simulink model "fangzhen20050606"  (Simulink 9.0)
settings: Solver=ode4  StartTime=0.0  StopTime=1200.0  FixedStep=0.05  RelTol=1e-3
InitFcn:
  | data
values from neighbouring files (symbols this model uses):
  A = [1    0     0 ... (first row only)    [cx.m]    (also in data.m = [Wex^2-W^2   Wex*Wey    Wex*Wez; data1.m = [Wex^2-W^2   Wex*Wey    Wex*Wez)
  a = F/m0    (= 0.2)    [data.m]    (also in data1.m = 0.02)
  a0 = 2*a*k/(4*a+k)    (= 0.08)    [data.m]    (also in data1.m = 0.00363636363636)
  AWcc = [1 1 1]*0.15/3600/3*pi/180    [data.m]    (also in data1.m)
  B = [   0    -2*Wez    2*Wey ... (first row only)    [data.m]    (also in data1.m)
  b = 0.00001*(a+a0)/(2*a*a0)    (= 8.75e-05)    [data.m]    (also in data1.m = 0.01625)
  c20 = -0.113    [data.m]    (also in data1.m)
  c22 = 0.0396    [data.m]    (also in data1.m)
  CWw = [1,1,1,1]*6e-5    [data.m]    (also in data1.m)
  d = 0.01    [data.m]    (also in data1.m = 0.1)
  DWN = [sin(bata)*cos(alpha)  sin(bata)*sin(alpha)  -sin(bata)*cos(alpha)  -sin(bata)*sin(alpha) ... (first row only)    [data.m]    (also in data1.m)
  F = 40    [data.m]    (also in data1.m = 4)
  f = f+2*pi    [E2C.m]    (also in data.m = -0.02; data1.m = 0.02)
  Gl = [-cos(xit0)*sin(fai0)   sin(xit0)*sin(fai0)    cos(fai0) ... (first row only)    [data.m]    (also in data1.m)
  HBd0 = IBd*We0    [data.m]    (also in data1.m)
  Hwmax = JW.*Wwmax    [data.m]    (also in data1.m)
  HWw0 = [0.01 0.01 0.01 0.01]    [data.m]    (also in data1.m)
  InvIBd = inv(IBd)    [data.m]    (also in data1.m)
  invJW = 1 ./JW    [data.m]    (also in data1.m)
  Isp = 300*9.8    (= 2940)    [data.m]    (also in data1.m)
  IW = [1,1,1,1]*1.e-6    [data.m]    (also in data1.m)
  JW = [1,1,1,1]*0.0017362    [data.m]    (also in data1.m)
  Kd = [19.2895;16.6643;22.1166]    [data.m]    (also in data1.m)
  Ki = [0.0503;0.0503;0.0503]    [data.m]    (also in data1.m)
  Kp = [7.0313;6.0484;8.0898]    [data.m]    (also in data1.m)
  m0 = 200    [data.m]    (also in data1.m)
  Mu = 4.794e3    (= 4794)    [data.m]    (also in data1.m)
  MWN = DWN'*inv(DWN*DWN')    [data.m]    (also in data1.m)
  Noise_gc = [1 -1 1]*6/3600*pi/180    [data.m]    (also in data1.m)
  Noise_gn = ([1 1 1]*0.0025/3.*pi/180).^2    [data.m]    (also in data1.m)
  Noise_rwn = ([1 1 1].*1e-10).^2    [data.m]    (also in data1.m)
  Qb0 = [QQQ(4);QQQ(1:3)]    [data.m]    (also in data1.m)
  r0 = [100;-200;1000]    [data.m]    (also in data1.m = [200;300;1000])
  R0 = Tl*[0;0;R0l]    [data.m]    (also in data1.m)
  re = 1750    [data.m]    (also in data1.m)
  rg0 = [3;-104;950]    [data.m]    (also in data1.m = [203;292;998])
  Rtb = [0;0;0]    [data.m]    (also in data1.m = [-30;50;0])
  T = 200    [data.m]    (also in data1.m = 1200)
  TA = [0 0 0]'    [data.m]    (also in data1.m)
  TB = [500 0 0]'    [data.m]    (also in data1.m)
  TC = [500 500 0]'    [data.m]    (also in data1.m)
  Tcmax = [1,1,1,1].*0.02    [data.m]    (also in data1.m)
  TWf0 = [1,1,1,1]*3e-4    [data.m]    (also in data1.m)
  v0 = [-0.1;0.1;-0.3]    [data.m]    (also in data1.m = [0.1;0.1;-1.0])
  vg0 = [0;-0.1;-0.4]    [data.m]    (also in data1.m = [0;-0.1;-0.7])
  Wcc = [1 1 1]*0.2    [data.m]    (also in data1.m)
  We = Tl*Gl'*[0;0;W]    [data.m]    (also in data1.m)
  Wgmax = 10*[1,1,1]'*pi/180    [data.m]    (also in data1.m)
undefined symbols (not defined in the file or in its folder): DiscIntNeverNeededParam, HB0, magnitude
libraries: sharedtransform x4, aerolibobsolete x4, sharedutil x1
(part 2 of 2)

== system fangzhen20050606/GNC System/轨迹制导0515(2)1/轨迹制导2/r ==
  tgo : Inport
  t : Inport  Port=2
  r0 : Inport  Port=3
  v0 : Inport  Port=4
  Gain1 : Gain  Gain=-2  SaturateOnIntegerOverflow=on  OutDataTypeStr=Inherit: Same as input  ParamDataTypeStr=Inherit: Same as input
  Gain2 : Gain  Gain=2  SaturateOnIntegerOverflow=on  OutDataTypeStr=Inherit: Same as input  ParamDataTypeStr=Inherit: Same as input
  Gain4 : Gain  Gain=-3  SaturateOnIntegerOverflow=on  OutDataTypeStr=Inherit: Same as input  ParamDataTypeStr=Inherit: Same as input
  Math Function1 : Math  Operator=magnitude^2  SaturateOnIntegerOverflow=on
  Math Function2 : Math  Operator=magnitude^2  SaturateOnIntegerOverflow=on
  Product{1..2,4,7..8} (5 alike) : Product  Inputs=**  SaturateOnIntegerOverflow=on  OutDataTypeStr=Inherit: Same as first input
  Product3 : Product  Inputs=**/  SaturateOnIntegerOverflow=on  OutDataTypeStr=Inherit: Same as first input
  Product6 : Product  Inputs=**/  SaturateOnIntegerOverflow=on  OutDataTypeStr=Inherit: Same as first input
  Sum1 : Sum  Inputs=++++  SaturateOnIntegerOverflow=on
  Sum2 : Sum  SaturateOnIntegerOverflow=on
  Sum3 : Sum  SaturateOnIntegerOverflow=on
  r : Outport
  wires:
  Product6/1 -> Sum1/2
  Product8/1 -> Product6/1
  Product7/1 -> Product6/3
  Sum3/1 -> Product6/2
  Product4/1 -> Sum3/1
  Gain2/1 -> Sum3/2
  Product3/1 -> Sum1/3
  Math Function1/1 -> Product8/2, Product3/1
  Sum2/1 -> Product3/2
  Math Function2/1 -> Product7/1, Product3/3
  Gain4/1 -> Sum2/2
  Gain1/1 -> Sum2/1
  Product2/1 -> Gain1/1
  tgo/1 -> Product7/2, Math Function2/1, Product4/2, Product2/2
  Product1/1 -> Sum1/1
  r0/1 -> Gain2/1, Sum1/4, Gain4/1
  v0/1 -> Product4/1, Product2/1, Product1/2
  t/1 -> Product8/1, Math Function1/1, Product1/1
  Sum1/1 -> r/1

== system fangzhen20050606/GNC System/轨迹制导0515(2)1/轨迹制导2/v ==
  tgo : Inport
  t : Inport  Port=2
  r0 : Inport  Port=3
  v0 : Inport  Port=4
  Gain1 : Gain  Gain=-6  SaturateOnIntegerOverflow=on  OutDataTypeStr=Inherit: Same as input  ParamDataTypeStr=Inherit: Same as input
  Gain2 : Gain  Gain=-4  SaturateOnIntegerOverflow=on  OutDataTypeStr=Inherit: Same as input  ParamDataTypeStr=Inherit: Same as input
  Gain4 : Gain  Gain=6  SaturateOnIntegerOverflow=on  OutDataTypeStr=Inherit: Same as input  ParamDataTypeStr=Inherit: Same as input
  Gain5 : Gain  Gain=3  SaturateOnIntegerOverflow=on  OutDataTypeStr=Inherit: Same as input  ParamDataTypeStr=Inherit: Same as input
  Math Function1 : Math  Operator=magnitude^2  SaturateOnIntegerOverflow=on
  Math Function4 : Math  Operator=magnitude^2  SaturateOnIntegerOverflow=on
  Product1 : Product  Inputs=**  SaturateOnIntegerOverflow=on  OutDataTypeStr=Inherit: Same as first input
  Product2 : Product  Inputs=**/  SaturateOnIntegerOverflow=on  OutDataTypeStr=Inherit: Same as first input
  Product5 : Product  Inputs=**/  SaturateOnIntegerOverflow=on  OutDataTypeStr=Inherit: Same as first input
  Product9 : Product  Inputs=**  SaturateOnIntegerOverflow=on  OutDataTypeStr=Inherit: Same as first input
  Sum1 : Sum  Inputs=+++  SaturateOnIntegerOverflow=on
  Sum2 : Sum  SaturateOnIntegerOverflow=on
  Sum3 : Sum  SaturateOnIntegerOverflow=on
  v : Outport
  wires:
  Product2/1 -> Sum1/1
  Product9/1 -> Product2/3
  Math Function1/1 -> Product2/1
  Sum3/1 -> Product2/2
  Gain4/1 -> Sum3/2
  Gain5/1 -> Sum3/1
  Product5/1 -> Sum1/2
  Math Function4/1 -> Product9/2, Product5/3
  t/1 -> Math Function1/1, Product5/1
  Sum2/1 -> Product5/2
  Gain2/1 -> Sum2/1
  Product1/1 -> Gain5/1, Gain2/1
  tgo/1 -> Product9/1, Math Function4/1, Product1/1
  Gain1/1 -> Sum2/2
  r0/1 -> Gain4/1, Gain1/1
  v0/1 -> Product1/2, Sum1/3
  Sum1/1 -> v/1

== system fangzhen20050606/GNC System/轨迹制导0515(2)1/轨迹制导4/C0 ==
  r : Inport
  v : Inport  Port=2
  tgo : Inport  Port=3
  rt : Inport  Port=4
  Gain : Gain  Gain=-6  SaturateOnIntegerOverflow=on  OutDataTypeStr=Inherit: Same as input  ParamDataTypeStr=Inherit: Same as input
  Gain1 : Gain  Gain=-12  SaturateOnIntegerOverflow=on  OutDataTypeStr=Inherit: Same as input  ParamDataTypeStr=Inherit: Same as input
  Math Function : Math  Operator=magnitude^2  SaturateOnIntegerOverflow=on
  Product : Product  Inputs=*/  SaturateOnIntegerOverflow=on  OutDataTypeStr=Inherit: Same as first input
  Product1 : Product  Inputs=*/  SaturateOnIntegerOverflow=on  OutDataTypeStr=Inherit: Same as first input
  Sum : Sum  SaturateOnIntegerOverflow=on
  Sum1 : Sum  Inputs=+-  SaturateOnIntegerOverflow=on
  C0 : Outport
  wires:
  tgo/1 -> Math Function/1, Product1/2
  v/1 -> Product1/1
  Product1/1 -> Gain/1
  Math Function/1 -> Product/2
  Product/1 -> Gain1/1
  Gain1/1 -> Sum/2
  Gain/1 -> Sum/1
  Sum/1 -> C0/1
  Sum1/1 -> Product/1
  r/1 -> Sum1/1
  rt/1 -> Sum1/2

== system fangzhen20050606/GNC System/轨迹制导0515(2)1/轨迹制导4/C1 ==
  r : Inport
  v : Inport  Port=2
  tgo : Inport  Port=3
  rt : Inport  Port=4
  Gain2 : Gain  Gain=18  SaturateOnIntegerOverflow=on  OutDataTypeStr=Inherit: Same as input  ParamDataTypeStr=Inherit: Same as input
  Gain3 : Gain  Gain=48  SaturateOnIntegerOverflow=on  OutDataTypeStr=Inherit: Same as input  ParamDataTypeStr=Inherit: Same as input
  Math Function1 : Math  Operator=magnitude^2  SaturateOnIntegerOverflow=on
  Product2 : Product  Inputs=*/  SaturateOnIntegerOverflow=on  OutDataTypeStr=Inherit: Same as first input
  Product3 : Product  Inputs=**  SaturateOnIntegerOverflow=on  OutDataTypeStr=Inherit: Same as first input
  Product4 : Product  Inputs=/*  SaturateOnIntegerOverflow=on  OutDataTypeStr=Inherit: Same as first input
  Sum1 : Sum  SaturateOnIntegerOverflow=on
  Sum2 : Sum  Inputs=+-  SaturateOnIntegerOverflow=on
  C1 : Outport
  wires:
  tgo/1 -> Math Function1/1, Product3/2
  Math Function1/1 -> Product2/2, Product3/1
  v/1 -> Product2/1
  Product2/1 -> Gain2/1
  Product3/1 -> Product4/1
  Product4/1 -> Gain3/1
  Sum1/1 -> C1/1
  Gain3/1 -> Sum1/2
  Gain2/1 -> Sum1/1
  Sum2/1 -> Product4/2
  r/1 -> Sum2/1
  rt/1 -> Sum2/2

== system fangzhen20050606/GNC System/轨迹制导0515(2)1/轨迹制导4/C2 ==
  r : Inport
  v : Inport  Port=2
  tgo : Inport  Port=3
  rt : Inport  Port=4
  Gain2 : Gain  Gain=-12  SaturateOnIntegerOverflow=on  OutDataTypeStr=Inherit: Same as input  ParamDataTypeStr=Inherit: Same as input
  Gain3 : Gain  Gain=-36  SaturateOnIntegerOverflow=on  OutDataTypeStr=Inherit: Same as input  ParamDataTypeStr=Inherit: Same as input
  Math Function1 : Math  Operator=magnitude^2  SaturateOnIntegerOverflow=on
  Product2 : Product  Inputs=*/  SaturateOnIntegerOverflow=on  OutDataTypeStr=Inherit: Same as first input
  Product3 : Product  Inputs=**  SaturateOnIntegerOverflow=on  OutDataTypeStr=Inherit: Same as first input
  Product4 : Product  Inputs=**  SaturateOnIntegerOverflow=on  OutDataTypeStr=Inherit: Same as first input
  Product5 : Product  Inputs=/*  SaturateOnIntegerOverflow=on  OutDataTypeStr=Inherit: Same as first input
  Sum1 : Sum  SaturateOnIntegerOverflow=on
  Sum2 : Sum  Inputs=+-  SaturateOnIntegerOverflow=on
  C2 : Outport
  wires:
  tgo/1 -> Math Function1/1, Product3/2
  Math Function1/1 -> Product3/1, Product4/1, Product4/2
  Product3/1 -> Product2/2
  v/1 -> Product2/1
  Product2/1 -> Gain2/1
  Product4/1 -> Product5/1
  Product5/1 -> Gain3/1
  Gain3/1 -> Sum1/2
  Gain2/1 -> Sum1/1
  Sum1/1 -> C2/1
  rt/1 -> Sum2/2
  Sum2/1 -> Product5/2
  r/1 -> Sum2/1

== system fangzhen20050606/GNC System/轨迹制导0515(2)1/轨迹制导4/r ==
  C0 : Inport
  C1 : Inport  Port=2
  C2 : Inport  Port=3
  t : Inport  Port=4
  r0 : Inport  Port=5
  v0 : Inport  Port=6
  Gain1 : Gain  Gain=0.5  SaturateOnIntegerOverflow=on  OutDataTypeStr=Inherit: Same as input  ParamDataTypeStr=Inherit: Same as input
  Gain2 : Gain  Gain=1/12  SaturateOnIntegerOverflow=on  OutDataTypeStr=Inherit: Same as input  ParamDataTypeStr=Inherit: Same as input
  Gain3 : Gain  Gain=1/6  SaturateOnIntegerOverflow=on  OutDataTypeStr=Inherit: Same as input  ParamDataTypeStr=Inherit: Same as input
  Math Function1 : Math  Operator=magnitude^2  SaturateOnIntegerOverflow=on
  Product{1..4,6..7} (6 alike) : Product  Inputs=**  SaturateOnIntegerOverflow=on  OutDataTypeStr=Inherit: Same as first input
  Sum1 : Sum  Inputs=+++++  SaturateOnIntegerOverflow=on
  r : Outport
  wires:
  t/1 -> Math Function1/1, Product2/2, Product7/1
  C0/1 -> Product3/1
  C1/1 -> Product1/1
  Product1/1 -> Gain3/1
  Math Function1/1 -> Product3/2, Product2/1, Product4/1, Product4/2
  Product3/1 -> Gain1/1
  Product2/1 -> Product1/2
  C2/1 -> Product6/1
  Product4/1 -> Product6/2
  Product6/1 -> Gain2/1
  v0/1 -> Product7/2
  Gain1/1 -> Sum1/1
  Gain3/1 -> Sum1/2
  Gain2/1 -> Sum1/3
  Product7/1 -> Sum1/4
  r0/1 -> Sum1/5
  Sum1/1 -> r/1

== system fangzhen20050606/GNC System/轨迹制导0515(2)1/轨迹制导4/v ==
  C0 : Inport
  C1 : Inport  Port=2
  C2 : Inport  Port=3
  t : Inport  Port=4
  v0 : Inport  Port=5
  Gain1 : Gain  Gain=1/3  SaturateOnIntegerOverflow=on  OutDataTypeStr=Inherit: Same as input  ParamDataTypeStr=Inherit: Same as input
  Gain3 : Gain  Gain=0.5  SaturateOnIntegerOverflow=on  OutDataTypeStr=Inherit: Same as input  ParamDataTypeStr=Inherit: Same as input
  Math Function1 : Math  Operator=magnitude^2  SaturateOnIntegerOverflow=on
  Product{1,3..5} (4 alike) : Product  Inputs=**  SaturateOnIntegerOverflow=on  OutDataTypeStr=Inherit: Same as first input
  Sum1 : Sum  Inputs=++++  SaturateOnIntegerOverflow=on
  v : Outport
  wires:
  C0/1 -> Product3/1
  t/1 -> Product3/2, Math Function1/1, Product5/2
  Math Function1/1 -> Product1/2, Product5/1
  C1/1 -> Product1/1
  Product1/1 -> Gain3/1
  C2/1 -> Product4/1
  Product5/1 -> Product4/2
  Product4/1 -> Gain1/1
  Product3/1 -> Sum1/1
  Gain3/1 -> Sum1/2
  Gain1/1 -> Sum1/3
  v0/1 -> Sum1/4
  Sum1/1 -> v/1

== system fangzhen20050606/Dynamics System动力系统/Attitude姿态/反作用飞轮/Torque/3x3 Cross Product ==
  A : Inport
  B : Inport  Port=2
  Product : Product  SaturateOnIntegerOverflow=on  InputSameDT=on  OutDataTypeStr=Inherit: Same as first input
  Product1 : Product  SaturateOnIntegerOverflow=on  InputSameDT=on  OutDataTypeStr=Inherit: Same as first input
  Selector : Selector  InputPortWidth=3  IndexOptions=Index vector (dialog)  Indices=[2 3 1]  OutputSizes=1
  Selector1 : Selector  InputPortWidth=3  IndexOptions=Index vector (dialog)  Indices=[3 1 2]  OutputSizes=1
  Selector2 : Selector  InputPortWidth=3  IndexOptions=Index vector (dialog)  Indices=[2 3 1]  OutputSizes=1
  Selector3 : Selector  InputPortWidth=3  IndexOptions=Index vector (dialog)  Indices=[3 1 2]  OutputSizes=1
  Sum : Sum  Inputs=+|-  SaturateOnIntegerOverflow=on  InputSameDT=on  OutDataTypeStr=Inherit: Same as first input
  C : Outport  InitialOutput=0
  wires:
  Sum/1 -> C/1
  B/1 -> Selector1/1, Selector2/1
  Selector/1 -> Product/1
  A/1 -> Selector/1, Selector3/1
  Product/1 -> Sum/1
  Selector1/1 -> Product/2
  Product1/1 -> Sum/2
  Selector2/1 -> Product1/2
  Selector3/1 -> Product1/1

== system fangzhen20050606/Dynamics System动力系统/Orbit轨道/轨道动力学模型/小行星引力加速度/小行星引力 ==
  note: z'
  note: y'
  note: x'
  r' : Inport
  Demux : Demux  Outputs=3
  K : Subsystem
  L : Subsystem
  Mux : Mux  Inputs=3
  Ux : Subsystem
  Uy : Subsystem
  Uz : Subsystem
  rt : Subsystem
  U : Outport
  wires:
  Demux/1 -> Ux/1(x'), L/2(x')
  r'/1 -> Demux/1, rt/1(r')
  Mux/1 -> U/1
  Uy/1(Uy) -> Mux/2
  Ux/1(Ux) -> Mux/1
  Uz/1(Uz) -> Mux/3
  rt/1(rt) -> Ux/2(rt), Uz/2(rt), K/2(rt), Uy/2(rt)
  Demux/3 -> Uz/1(z'), K/1(z')
  Demux/2 -> Uy/1(y'), L/1(y')
  K/1(K) -> Uz/4(K), Ux/4(K), Uy/4(K)
  L/1(L) -> Uz/3(L), Ux/3(L), Uy/3(L)

== system fangzhen20050606/GNC System/导航与滤波/Calculate/Subsystem3/e2 ==
  A : Inport
  B : Inport  Port=2
  Product : Product  SaturateOnIntegerOverflow=on  InputSameDT=on  OutDataTypeStr=Inherit: Same as first input
  Product1 : Product  SaturateOnIntegerOverflow=on  InputSameDT=on  OutDataTypeStr=Inherit: Same as first input
  Selector : Selector  InputPortWidth=3  IndexOptions=Index vector (dialog)  Indices=[2 3 1]  OutputSizes=1
  Selector1 : Selector  InputPortWidth=3  IndexOptions=Index vector (dialog)  Indices=[3 1 2]  OutputSizes=1
  Selector2 : Selector  InputPortWidth=3  IndexOptions=Index vector (dialog)  Indices=[2 3 1]  OutputSizes=1
  Selector3 : Selector  InputPortWidth=3  IndexOptions=Index vector (dialog)  Indices=[3 1 2]  OutputSizes=1
  Sum : Sum  Inputs=+|-  SaturateOnIntegerOverflow=on  InputSameDT=on  OutDataTypeStr=Inherit: Same as first input
  C : Outport  InitialOutput=0
  wires:
  Sum/1 -> C/1
  B/1 -> Selector1/1, Selector2/1
  Selector/1 -> Product/1
  A/1 -> Selector/1, Selector3/1
  Product/1 -> Sum/1
  Selector1/1 -> Product/2
  Product1/1 -> Sum/2
  Selector2/1 -> Product1/2
  Selector3/1 -> Product1/1

== system fangzhen20050606/GNC System/导航与滤波/Calculate/Subsystem3/e4 ==
  A : Inport
  B : Inport  Port=2
  Product : Product  SaturateOnIntegerOverflow=on  InputSameDT=on  OutDataTypeStr=Inherit: Same as first input
  Product1 : Product  SaturateOnIntegerOverflow=on  InputSameDT=on  OutDataTypeStr=Inherit: Same as first input
  Selector : Selector  InputPortWidth=3  IndexOptions=Index vector (dialog)  Indices=[2 3 1]  OutputSizes=1
  Selector1 : Selector  InputPortWidth=3  IndexOptions=Index vector (dialog)  Indices=[3 1 2]  OutputSizes=1
  Selector2 : Selector  InputPortWidth=3  IndexOptions=Index vector (dialog)  Indices=[2 3 1]  OutputSizes=1
  Selector3 : Selector  InputPortWidth=3  IndexOptions=Index vector (dialog)  Indices=[3 1 2]  OutputSizes=1
  Sum : Sum  Inputs=+|-  SaturateOnIntegerOverflow=on  InputSameDT=on  OutDataTypeStr=Inherit: Same as first input
  C : Outport  InitialOutput=0
  wires:
  Selector3/1 -> Product1/1
  Selector2/1 -> Product1/2
  Product1/1 -> Sum/2
  Selector1/1 -> Product/2
  Product/1 -> Sum/1
  A/1 -> Selector3/1, Selector/1
  Selector/1 -> Product/1
  B/1 -> Selector2/1, Selector1/1
  Sum/1 -> C/1

== system fangzhen20050606/Dynamics System动力系统/Orbit轨道/轨道动力学模型/小行星引力加速度/小行星引力/K ==
  z' : Inport
  rt : Inport  Port=2
  Product : Product  Inputs=*/  SaturateOnIntegerOverflow=on  OutDataTypeStr=Inherit: Same as first input
  Trigonometric Function : Trigonometry  Operator=asin
  K : Outport
  wires:
  Trigonometric Function/1 -> K/1
  z'/1 -> Product/1
  rt/1 -> Product/2
  Product/1 -> Trigonometric Function/1

== system fangzhen20050606/Dynamics System动力系统/Orbit轨道/轨道动力学模型/小行星引力加速度/小行星引力/L ==
  y' : Inport
  x' : Inport  Port=2
  Product : Product  Inputs=*/  SaturateOnIntegerOverflow=on  OutDataTypeStr=Inherit: Same as first input
  Trigonometric Function : Trigonometry  Operator=atan
  L : Outport
  wires:
  Product/1 -> Trigonometric Function/1
  y'/1 -> Product/1
  x'/1 -> Product/2
  Trigonometric Function/1 -> L/1

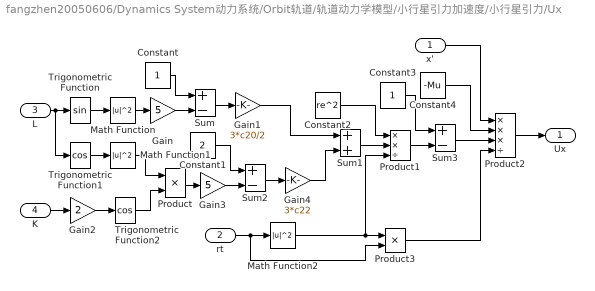
== system fangzhen20050606/Dynamics System动力系统/Orbit轨道/轨道动力学模型/小行星引力加速度/小行星引力/Ux ==
  x' : Inport
  rt : Inport  Port=2
  L : Inport  Port=3
  K : Inport  Port=4
  Constant : Constant
  Constant1 : Constant  Value=2
  Constant2 : Constant  Value=re^2
  Constant3 : Constant
  Constant4 : Constant  Value=-Mu
  Gain : Gain  Gain=5  SaturateOnIntegerOverflow=on  OutDataTypeStr=Inherit: Same as input  ParamDataTypeStr=Inherit: Same as input
  Gain1 : Gain  Gain=3*c20/2  SaturateOnIntegerOverflow=on  OutDataTypeStr=Inherit: Same as input  ParamDataTypeStr=Inherit: Same as input
  Gain2 : Gain  Gain=2  SaturateOnIntegerOverflow=on  OutDataTypeStr=Inherit: Same as input  ParamDataTypeStr=Inherit: Same as input
  Gain3 : Gain  Gain=5  SaturateOnIntegerOverflow=on  OutDataTypeStr=Inherit: Same as input  ParamDataTypeStr=Inherit: Same as input
  Gain4 : Gain  Gain=3*c22  SaturateOnIntegerOverflow=on  OutDataTypeStr=Inherit: Same as input  ParamDataTypeStr=Inherit: Same as input
  Math Function : Math  Operator=magnitude^2  SaturateOnIntegerOverflow=on
  Math Function1 : Math  Operator=magnitude^2  SaturateOnIntegerOverflow=on
  Math Function2 : Math  Operator=magnitude^2  SaturateOnIntegerOverflow=on
  Product : Product  SaturateOnIntegerOverflow=on  OutDataTypeStr=Inherit: Same as first input
  Product1 : Product  Inputs=**/  SaturateOnIntegerOverflow=on  OutDataTypeStr=Inherit: Same as first input
  Product2 : Product  Inputs=***/  SaturateOnIntegerOverflow=on  OutDataTypeStr=Inherit: Same as first input
  Product3 : Product  SaturateOnIntegerOverflow=on  OutDataTypeStr=Inherit: Same as first input
  Sum : Sum  Inputs=+-  SaturateOnIntegerOverflow=on
  Sum1 : Sum  SaturateOnIntegerOverflow=on
  Sum2 : Sum  Inputs=+-  SaturateOnIntegerOverflow=on
  Sum3 : Sum  Inputs=+-  SaturateOnIntegerOverflow=on
  Trigonometric Function : Trigonometry
  Trigonometric Function1 : Trigonometry  Operator=cos
  Trigonometric Function2 : Trigonometry  Operator=cos
  Ux : Outport
  wires:
  L/1 -> Trigonometric Function/1, Trigonometric Function1/1
  Trigonometric Function/1 -> Math Function/1
  Math Function/1 -> Gain/1
  Constant/1 -> Sum/1
  Gain/1 -> Sum/2
  Sum/1 -> Gain1/1
  Trigonometric Function1/1 -> Math Function1/1
  K/1 -> Gain2/1
  Gain2/1 -> Trigonometric Function2/1
  Trigonometric Function2/1 -> Product/2
  Math Function1/1 -> Product/1
  Product/1 -> Gain3/1
  Constant1/1 -> Sum2/1
  Gain3/1 -> Sum2/2
  Sum2/1 -> Gain4/1
  Gain4/1 -> Sum1/2
  Gain1/1 -> Sum1/1
  rt/1 -> Math Function2/1, Product3/2
  Sum1/1 -> Product1/2
  Math Function2/1 -> Product1/3, Product3/1
  Constant2/1 -> Product1/1
  Product1/1 -> Sum3/2
  Constant3/1 -> Sum3/1
  Sum3/1 -> Product2/3
  Constant4/1 -> Product2/2
  x'/1 -> Product2/1
  Product3/1 -> Product2/4
  Product2/1 -> Ux/1

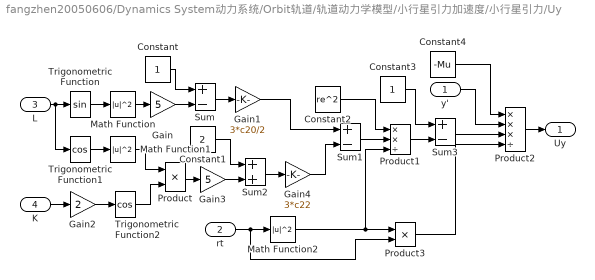
== system fangzhen20050606/Dynamics System动力系统/Orbit轨道/轨道动力学模型/小行星引力加速度/小行星引力/Uy ==
  y' : Inport
  rt : Inport  Port=2
  L : Inport  Port=3
  K : Inport  Port=4
  Constant : Constant
  Constant1 : Constant  Value=2
  Constant2 : Constant  Value=re^2
  Constant3 : Constant
  Constant4 : Constant  Value=-Mu
  Gain : Gain  Gain=5  SaturateOnIntegerOverflow=on  OutDataTypeStr=Inherit: Same as input  ParamDataTypeStr=Inherit: Same as input
  Gain1 : Gain  Gain=3*c20/2  SaturateOnIntegerOverflow=on  OutDataTypeStr=Inherit: Same as input  ParamDataTypeStr=Inherit: Same as input
  Gain2 : Gain  Gain=2  SaturateOnIntegerOverflow=on  OutDataTypeStr=Inherit: Same as input  ParamDataTypeStr=Inherit: Same as input
  Gain3 : Gain  Gain=5  SaturateOnIntegerOverflow=on  OutDataTypeStr=Inherit: Same as input  ParamDataTypeStr=Inherit: Same as input
  Gain4 : Gain  Gain=3*c22  SaturateOnIntegerOverflow=on  OutDataTypeStr=Inherit: Same as input  ParamDataTypeStr=Inherit: Same as input
  Math Function : Math  Operator=magnitude^2  SaturateOnIntegerOverflow=on
  Math Function1 : Math  Operator=magnitude^2  SaturateOnIntegerOverflow=on
  Math Function2 : Math  Operator=magnitude^2  SaturateOnIntegerOverflow=on
  Product : Product  SaturateOnIntegerOverflow=on  OutDataTypeStr=Inherit: Same as first input
  Product1 : Product  Inputs=**/  SaturateOnIntegerOverflow=on  OutDataTypeStr=Inherit: Same as first input
  Product2 : Product  Inputs=***/  SaturateOnIntegerOverflow=on  OutDataTypeStr=Inherit: Same as first input
  Product3 : Product  SaturateOnIntegerOverflow=on  OutDataTypeStr=Inherit: Same as first input
  Sum : Sum  Inputs=+-  SaturateOnIntegerOverflow=on
  Sum1 : Sum  Inputs=+-  SaturateOnIntegerOverflow=on
  Sum2 : Sum  SaturateOnIntegerOverflow=on
  Sum3 : Sum  Inputs=+-  SaturateOnIntegerOverflow=on
  Trigonometric Function : Trigonometry
  Trigonometric Function1 : Trigonometry  Operator=cos
  Trigonometric Function2 : Trigonometry  Operator=cos
  Uy : Outport
  wires:
  L/1 -> Trigonometric Function/1, Trigonometric Function1/1
  Trigonometric Function/1 -> Math Function/1
  Math Function/1 -> Gain/1
  Constant/1 -> Sum/1
  Gain/1 -> Sum/2
  Sum/1 -> Gain1/1
  Trigonometric Function1/1 -> Math Function1/1
  K/1 -> Gain2/1
  Gain2/1 -> Trigonometric Function2/1
  Trigonometric Function2/1 -> Product/2
  Math Function1/1 -> Product/1
  Product/1 -> Gain3/1
  Constant1/1 -> Sum2/1
  Gain3/1 -> Sum2/2
  Sum2/1 -> Gain4/1
  Gain4/1 -> Sum1/2
  Gain1/1 -> Sum1/1
  rt/1 -> Math Function2/1, Product3/2
  Sum1/1 -> Product1/2
  Math Function2/1 -> Product1/3, Product3/1
  Constant2/1 -> Product1/1
  Product1/1 -> Sum3/2
  Constant3/1 -> Sum3/1
  Product2/1 -> Uy/1
  y'/1 -> Product2/2
  Constant4/1 -> Product2/1
  Sum3/1 -> Product2/3
  Product3/1 -> Product2/4

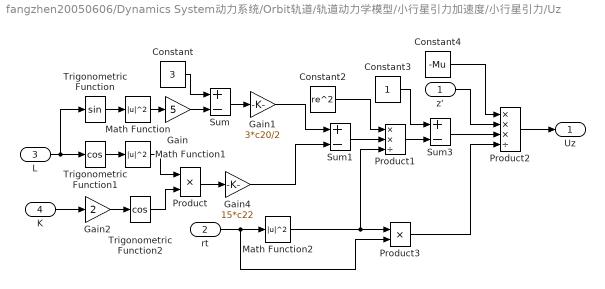
== system fangzhen20050606/Dynamics System动力系统/Orbit轨道/轨道动力学模型/小行星引力加速度/小行星引力/Uz ==
  z' : Inport
  rt : Inport  Port=2
  L : Inport  Port=3
  K : Inport  Port=4
  Constant : Constant  Value=3
  Constant2 : Constant  Value=re^2
  Constant3 : Constant
  Constant4 : Constant  Value=-Mu
  Gain : Gain  Gain=5  SaturateOnIntegerOverflow=on  OutDataTypeStr=Inherit: Same as input  ParamDataTypeStr=Inherit: Same as input
  Gain1 : Gain  Gain=3*c20/2  SaturateOnIntegerOverflow=on  OutDataTypeStr=Inherit: Same as input  ParamDataTypeStr=Inherit: Same as input
  Gain2 : Gain  Gain=2  SaturateOnIntegerOverflow=on  OutDataTypeStr=Inherit: Same as input  ParamDataTypeStr=Inherit: Same as input
  Gain4 : Gain  Gain=15*c22  SaturateOnIntegerOverflow=on  OutDataTypeStr=Inherit: Same as input  ParamDataTypeStr=Inherit: Same as input
  Math Function : Math  Operator=magnitude^2  SaturateOnIntegerOverflow=on
  Math Function1 : Math  Operator=magnitude^2  SaturateOnIntegerOverflow=on
  Math Function2 : Math  Operator=magnitude^2  SaturateOnIntegerOverflow=on
  Product : Product  SaturateOnIntegerOverflow=on  OutDataTypeStr=Inherit: Same as first input
  Product1 : Product  Inputs=**/  SaturateOnIntegerOverflow=on  OutDataTypeStr=Inherit: Same as first input
  Product2 : Product  Inputs=***/  SaturateOnIntegerOverflow=on  OutDataTypeStr=Inherit: Same as first input
  Product3 : Product  SaturateOnIntegerOverflow=on  OutDataTypeStr=Inherit: Same as first input
  Sum : Sum  Inputs=+-  SaturateOnIntegerOverflow=on
  Sum1 : Sum  Inputs=+-  SaturateOnIntegerOverflow=on
  Sum3 : Sum  Inputs=+-  SaturateOnIntegerOverflow=on
  Trigonometric Function : Trigonometry
  Trigonometric Function1 : Trigonometry  Operator=cos
  Trigonometric Function2 : Trigonometry  Operator=cos
  Uz : Outport
  wires:
  Trigonometric Function/1 -> Math Function/1
  Math Function/1 -> Gain/1
  Constant/1 -> Sum/1
  Gain/1 -> Sum/2
  Sum/1 -> Gain1/1
  Trigonometric Function1/1 -> Math Function1/1
  Gain2/1 -> Trigonometric Function2/1
  Trigonometric Function2/1 -> Product/2
  Math Function1/1 -> Product/1
  Product/1 -> Gain4/1
  Gain1/1 -> Sum1/1
  rt/1 -> Math Function2/1, Product3/2
  Sum1/1 -> Product1/2
  Math Function2/1 -> Product1/3, Product3/1
  Constant2/1 -> Product1/1
  Product1/1 -> Sum3/2
  Constant3/1 -> Sum3/1
  z'/1 -> Product2/2
  Constant4/1 -> Product2/1
  Sum3/1 -> Product2/3
  Product3/1 -> Product2/4
  K/1 -> Gain2/1
  L/1 -> Trigonometric Function1/1, Trigonometric Function/1
  Gain4/1 -> Sum1/2
  Product2/1 -> Uz/1

== system fangzhen20050606/Dynamics System动力系统/Orbit轨道/轨道动力学模型/小行星引力加速度/小行星引力/rt ==
  r' : Inport
  Demux : Demux  Outputs=3
  Math Function : Math  Operator=sqrt  SaturateOnIntegerOverflow=on
  Math Function1 : Math  Operator=magnitude^2  SaturateOnIntegerOverflow=on
  Math Function2 : Math  Operator=magnitude^2  SaturateOnIntegerOverflow=on
  Math Function3 : Math  Operator=magnitude^2  SaturateOnIntegerOverflow=on
  Sum : Sum  Inputs=+++  SaturateOnIntegerOverflow=on
  rt : Outport
  wires:
  r'/1 -> Demux/1
  Demux/1 -> Math Function1/1
  Demux/2 -> Math Function2/1
  Demux/3 -> Math Function3/1
  Math Function/1 -> rt/1
  Sum/1 -> Math Function/1
  Math Function1/1 -> Sum/1
  Math Function2/1 -> Sum/2
  Math Function3/1 -> Sum/3
